simulink model "PD_digital"  (R2017b)
settings: Solver=VariableStepAuto  StartTime=0.0  StopTime=7  RelTol=1e-3
settings Model: Creator=fernandopassold  LastModifiedBy=fernandopassold

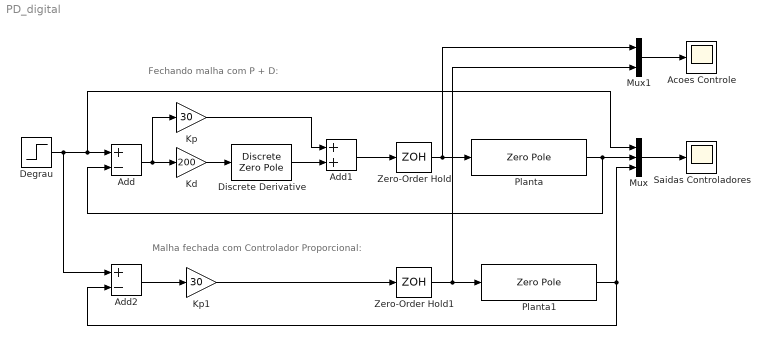
== system PD_digital ==
  note: Fechando malha com P + D:
  note: Malha fechada com Controlador Proporcional:
  Acoes Controle : Scope
  Add : Sum  Inputs=+-
  Add1 : Sum
  Add2 : Sum  Inputs=+-
  Degrau : Step  SampleTime=0
  Discrete Derivative : DiscreteZeroPole  Poles=[0]  Gain=1  SampleTime=0.1
  Kd : Gain  Gain=200
  Kp : Gain  Gain=30
  Kp1 : Gain  Gain=30
  Mux : Mux  Inputs=3
  Mux1 : Mux  Inputs=2
  Planta : ZeroPole  Zeros=[ ]  Poles=[-1 -2 -10]
  Planta1 : ZeroPole  Zeros=[ ]  Poles=[-1 -2 -10]
  Saidas Controladores : Scope
  Zero-Order Hold : ZeroOrderHold  SampleTime=0.1
  Zero-Order Hold1 : ZeroOrderHold  SampleTime=0.1
  wires:
  Planta/1 -> Add/2, Mux/2
  Zero-Order Hold/1 -> Mux1/1, Planta/1
  Add/1 -> Kd/1, Kp/1
  Discrete Derivative/1 -> Add1/2
  Add1/1 -> Zero-Order Hold/1
  Kp/1 -> Add1/1
  Zero-Order Hold1/1 -> Mux1/2, Planta1/1
  Add2/1 -> Kp1/1
  Degrau/1 -> Add2/1, Mux/1, Add/1
  Kp1/1 -> Zero-Order Hold1/1
  Mux/1 -> Saidas Controladores/1
  Planta1/1 -> Add2/2, Mux/3
  Kd/1 -> Discrete Derivative/1
  Mux1/1 -> Acoes Controle/1
